simulink model "s_proz2"  (Simulink 4.00)
settings: Solver=ode45  SolverMode=SingleTasking  StartTime=0.0  StopTime=999999  MaxStep=10  RelTol=1e-3  AbsTol=1e-6
settings Model: LastModifiedBy=Administrator  SaveTime=off  SaveOutput=off  LimitDataPoints=off  BlockReductionOpt=off

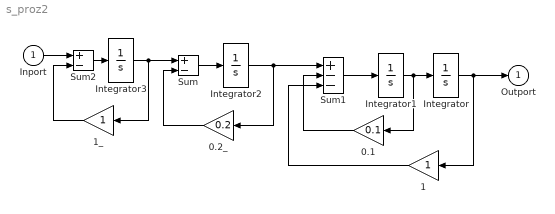
== system s_proz2 ==
  Inport : Inport  Port=1
  0.1 : Gain  Orientation=left  Gain=0.1  Multiplication=Element-wise(K.*u)  SaturateOnIntegerOverflow=on
  0.2_ : Gain  Orientation=left  Gain=0.2  Multiplication=Element-wise(K.*u)  SaturateOnIntegerOverflow=on
  1 : Gain  Orientation=left  Gain=1  Multiplication=Element-wise(K.*u)  SaturateOnIntegerOverflow=on
  1_ : Gain  Orientation=left  Gain=1  Multiplication=Element-wise(K.*u)  SaturateOnIntegerOverflow=on
  Integrator{,1..3} (4 alike) : Integrator  ExternalReset=none  InitialConditionSource=internal  InitialCondition=0  LimitOutput=off  UpperSaturationLimit=inf  LowerSaturationLimit=-inf  ShowSaturationPort=off  ShowStatePort=off  AbsoluteTolerance=auto
  Sum : Sum  Inputs=+-  SaturateOnIntegerOverflow=on
  Sum1 : Sum  Inputs=+--  SaturateOnIntegerOverflow=on
  Sum2 : Sum  Inputs=+-  SaturateOnIntegerOverflow=on
  Outport : Outport  Port=1  InitialOutput=0
  wires:
  1_/1 -> Sum2/2
  Integrator3/1 -> 1_/1, Sum/1
  Inport/1 -> Sum2/1
  Sum2/1 -> Integrator3/1
  Integrator/1 -> Outport/1, 1/1
  0.2_/1 -> Sum/2
  Integrator2/1 -> 0.2_/1, Sum1/1
  Sum/1 -> Integrator2/1
  1/1 -> Sum1/3
  0.1/1 -> Sum1/2
  Integrator1/1 -> 0.1/1, Integrator/1
  Sum1/1 -> Integrator1/1
